simulink model "Model_6DOF_B3"  (R2020b)
settings: Solver=FixedStepAuto  StartTime=0.0  StopTime=120  FixedStep=0.05  RelTol=1e-3
values from neighbouring files (symbols this model uses):
  Ba_0 = [0 0 0 0 0 0]    [ctrl_mode_param.m]
  Bb = 4418825.3321    [load_data.m]
  Bv_0 = [tgt_speed 0 0 0 0 0]    [ctrl_mode_param.m]
  Bx_0 = [0 0 tgt_depth 0 0 0]    [ctrl_mode_param.m]
  Ixx = 5.23e7    (= 52300000)    [load_data.m]
  Ixy = 0    [load_data.m]
  Ixz = 0    [load_data.m]
  Iyy = 1.375e9    (= 1375000000)    [load_data.m]
  Iyz = 0    [load_data.m]
  Izz = 1.367e9    (= 1367000000)    [load_data.m]
  Mb = 4418825.3321    [load_data.m]
  Xb = 0    [load_data.m]
  Xg = 0    [load_data.m]
  Yb = 0    [load_data.m]
  Yg = 0    [load_data.m]
  Zb = 0.4406    [load_data.m]
  Zg = 0    [load_data.m]
undefined symbols (not defined in the file or in its folder): dA_BP1, dA_BP2, dA_Hull, dA_PH, dA_Sail, dA_SProot, dA_X1a, dA_X1b, dA_X2a, dA_X2b, dA_X3a, dA_X3b, dA_X4a, dA_X4b, its, n_BP1, n_BP2, n_Hull, n_PH, n_Sail, n_SProot, n_X1a, n_X1b, n_X2a, n_X2b, n_X3a, n_X3b, n_X4a, n_X4b, nt_BP1, nt_BP2, nt_Hull, nt_PH, nt_Sail, nt_SProot, nt_X1a, nt_X1b, nt_X2a, nt_X2b, nt_X3a, nt_X3b, nt_X4a, nt_X4b, Usp, vt1_BP1, vt1_BP2, vt1_Hull, vt1_PH, vt1_Sail, vt1_SProot, vt1_X1a, vt1_X1b, vt1_X2a, vt1_X2b, vt1_X3a, vt1_X3b, vt1_X4a, vt1_X4b, vt2_BP1, vt2_BP2 ... (+27)
libraries: simulink x5
(part 2 of 15)

== system Model_6DOF_B3/HDM 6DOF V1/M 6d org ==
  Bx : Inport
  Bv : Inport  Port=2
  Ba : Inport  Port=3
  Alpha : Inport  Port=4
  Umag : Inport  Port=5
  dX : Inport  Port=6
  UeX : Inport  Port=7
  dLCG : Inport  Port=8
  dmass : Inport  Port=9
  Mvm : Inport  Port=10
  M'prop : Lookup_n-D  NumberOfTableDimensions=1  BreakpointsForDimension1=[-7.7166666 -5.1444444 -3.08666664]  Table=[-0.00022 -0.0002 -0.00015]  InternalRulePriority=Speed  RndMeth=Simplest  InputSameDT=on
  M'uvw : Lookup_n-D  NumberOfTableDimensions=3  BreakpointsForDimension1=|  BreakpointsForDimension2=|  BreakpointsForDimension3=|  Table=|  InternalRulePriority=Speed  RndMeth=Simplest  InputSameDT=on
      BreakpointsForDimension1=|
      | [-12
      | -8
      | -4
      | 0
      | 4
      | 8
      | 12]
      BreakpointsForDimension2=|
      | [-5.1444E+00
      | -3.0866E+00
      | -1.5433E+00
      | ]
      Table=|
      | reshape([-2.40251E-03
      | -1.59538E-03
      | -8.21748E-04
      | -3.60182E-06
      | 8.13350E-04
      | 1.50586E-03
      | 2.39707E-03
      | -2.43392E-03
      | -1.61509E-03
      | -8.50748E-04
      | -3.60182E-06
      | 8.24271E-04
      | 1.51842E-03
      | 2.43805E-03
      | -2.45014E-03
      | -1.65711E-03
      | -9.11210E-04
      | -3.60182E-06
      | 8.61300E-04
      | 1.57459E-03
      | 2.42777E-03
      | -2.54380E-03
      | -1.68842E-03
      | -8.33041E-04
      | 2.23377E-05
      | 8.77717E-04
      | 1.73310E-03
      | 2.58847E-03
      | -2.63734E-03
      | -1.75078E-03
      | -8.64221E-04
      | 2.23377E-05
      | 9.08896E-04
      | 1.79546E-03
      | 2.68201E-03
      | -2.83738E-03
      | -1.88414E-03
      | -9.30902E-04
      | 2.23377E-05
      | 9.75577E-04
      | 1.92882E-03
      | 2.88206E-03
      | -2.63786E-03
      | -1.74504E-03
      | -8.52211E-04
      | 4.06140E-05
      | 9.33439E-04
      | 1.82626E-03
      | 2.71909E-03
      | -2.63728E-03
      | -1.74465E-03
      | -8.52017E-04
      | 4.06140E-05
      | 9.33245E-04
      | 1.82588E-03
      | 2.71851E-03
      | -2.86138E-03
      | -1.89405E-03
      | -9.26716E-04
      | 4.06140E-05
      | 1.00794E-03
      | 1.97527E-03
      | 2.94260E-03
      | -0.002723494
      | -0.001792522
      | -0.000861549
      | 6.9423E-05
      | 0.001000396
      | 0.001931368
      | 0.002862341
      | -0.002736476
      | -0.001798489
      | -0.000860502
      | 6.9423E-05
      | 0.001015473
      | 0.00195346
      | 0.002891447
      | -0.002765582
      | -0.00182058
      | -0.000875579
      | 6.9423E-05
      | 0.001014425
      | 0.001959426
      | 0.002904428],[7,3,4])
      BreakpointsForDimension3=|
      | [-35.0624 -18.3724 -15.3724 -13.8724
      | ]
      settings: InputPortMap=u0,u1,u2
  MATLAB Function2 : MATLAB Function  TreatAsAtomicUnit=on
  Mdxi : Subsystem
  Mqq2 : Lookup_n-D  NumberOfTableDimensions=1  BreakpointsForDimension1=|  Table=|  InternalRulePriority=Speed  RndMeth=Simplest  InputSameDT=on
      BreakpointsForDimension1=|
      | [-0.02
      | -0.015
      | -0.012958963
      | -0.009719222
      | -0.006479482
      | -0.003239741
      | -0.00161987
      | -0.000647948
      | 0.000647948
      | 0.00161987
      | 0.003239741
      | 0.006479482
      | 0.009719222
      | 0.012958963
      | 0.015
      | 0.02
      | ]
      Table=|
      | [-2.2571E-03
      | -2.3029E-03
      | -2.0965E-03
      | -2.0229E-03
      | -2.1546E-03
      | -1.4789E-03
      | -1.5664E-03
      | -1.4544E-03
      | -1.4705E-03
      | -1.4942E-03
      | -1.8790E-03
      | -1.8821E-03
      | -2.1009E-03
      | -2.0521E-03
      | -2.1685E-03
      | -2.0822E-03
      | ]
  Muq : Lookup_n-D  BreakpointsForDimension1=|  BreakpointsForDimension2=|  Table=|  InternalRulePriority=Speed  RndMeth=Simplest  InputSameDT=on
      BreakpointsForDimension1=|
      | [-2.00E-01
      | -1.50E-01
      | -1.00E-01
      | -5.00E-02
      | 0.00E+00
      | 5.00E-02
      | 1.00E-01
      | 1.50E-01
      | 2.00E-01
      | ]
      Table=|
      | reshape([-3.95902E-04
      | -2.96922E-04
      | -1.97952E-04
      | -9.89720E-05
      | 0.00000E+00
      | 9.89750E-05
      | 1.97948E-04
      | 2.96928E-04
      | 3.95898E-04
      | -4.94864E-04
      | -3.71144E-04
      | -2.47434E-04
      | -1.23714E-04
      | 0.00000E+00
      | 1.23715E-04
      | 2.47426E-04
      | 3.71146E-04
      | 4.94856E-04
      | -5.69298E-04
      | -4.26978E-04
      | -2.84648E-04
      | -1.42328E-04
      | 0.00000E+00
      | 1.42322E-04
      | 2.84652E-04
      | 4.26972E-04
      | 5.69302E-04
      | -5.60922E-04
      | -4.20692E-04
      | -2.80462E-04
      | -1.40232E-04
      | 0.00000E+00
      | 1.40228E-04
      | 2.80458E-04
      | 4.20688E-04
      | 5.60918E-04],[9,4])
      BreakpointsForDimension2=|
      | [-7.7166 -5.1444 -3.08664 -1.54332
      | ]
      settings: InputPortMap=u0,u1
  Mwq : Lookup_n-D  NumberOfTableDimensions=1  BreakpointsForDimension1=|  Table=|  InternalRulePriority=Speed  RndMeth=Simplest  InputSameDT=on
      BreakpointsForDimension1=|
      | [-0.0015
      | -0.0012
      | -0.0009
      | -0.0006
      | -0.0003
      | -0.0001
      | 0.0001
      | 0.0003
      | 0.0006
      | 0.0009
      | 0.0012
      | 0.0015]
      Table=|
      | [-1.3011E-02
      | -1.6962E-02
      | -2.0682E-02
      | -3.1419E-02
      | -6.4407E-02
      | -1.9322E-01
      | 1.9322E-01
      | 6.4378E-02
      | 3.1944E-02
      | 2.1072E-02
      | 1.6415E-02
      | 1.3407E-02]
  My : MATLAB Function  TreatAsAtomicUnit=on
  Product4 : Product
  Product5 : Product
  Saturation2 : Saturate  UpperLimit=0.0015  LowerLimit=-0.0015
  Saturation3 : Saturate  UpperLimit=0.02  LowerLimit=-0.02
  Selector10 : Selector  InputPortWidth=6  IndexOptions=Index vector (dialog)  Indices=1  OutputSizes=1
  Selector2 : Selector  InputPortWidth=6  IndexOptions=Index vector (dialog)  Indices=3  OutputSizes=1
  Selector4 : Selector  InputPortWidth=6  IndexOptions=Index vector (dialog)  Indices=5  OutputSizes=1
  Selector8 : Selector  InputPortWidth=6  IndexOptions=Index vector (dialog)  Indices=3  OutputSizes=1
  To Workspace : ToWorkspace  VariableName=MApp  SaveFormat=Timeseries  SampleTime=-1
  To Workspace1 : ToWorkspace  VariableName=MStat  SaveFormat=Timeseries  SampleTime=-1
  To Workspace2 : ToWorkspace  VariableName=MHull  SaveFormat=Timeseries  SampleTime=-1
  To Workspace3 : ToWorkspace  VariableName=Mprop  SaveFormat=Timeseries  SampleTime=-1
  To Workspace4 : ToWorkspace  VariableName=Mtotal  SaveFormat=Timeseries  SampleTime=-1
  M : Outport
  wires:
  Bv/1 -> Selector10/1, Selector4/1, Selector8/1, My/2(Bv)
  Bx/1 -> My/1(Bx), Selector2/1
  Selector10/1 -> Muq/2, Product4/1, M'uvw/2, M'prop/1
  Ba/1 -> My/3(Ba)
  M'prop/1 -> My/7(Mprop)
  UeX/1 -> My/10(UeX)
  Selector4/1 -> MATLAB Function2/1(u), Saturation3/1, Product4/2
  Alpha/1 -> M'uvw/1
  Umag/1 -> My/9(Umag)
  dLCG/1 -> My/11(dLCG)
  dmass/1 -> My/12(dmass)
  dX/1 -> Mdxi/1(dX)
  Mqq2/1 -> My/4(Mqq)
  Mwq/1 -> My/5(Mwq)
  Product4/1 -> Muq/1
  Product5/1 -> Saturation2/1
  Selector8/1 -> Product5/2
  MATLAB Function2/1(y) -> Product5/1
  Saturation2/1 -> Mwq/1
  Saturation3/1 -> Mqq2/1
  Muq/1 -> My/6(Muq)
  My/1(MY) -> To Workspace4/1, M/1
  Mdxi/1(MdX) -> My/13(MdXi)
  Mvm/1 -> My/14(Mvm)
  Selector2/1 -> M'uvw/3, Mdxi/2(z)
  M'uvw/1 -> My/8(Muvw)
  My/2(MYApp) -> To Workspace/1
  My/3(MYStat) -> To Workspace1/1
  My/5(MYprop) -> To Workspace3/1
  My/4(MYhull) -> To Workspace2/1

== system Model_6DOF_B3/HDM 6DOF V1/N ==
  Bx : Inport
  Bv : Inport  Port=2
  Ba : Inport  Port=3
  Beta : Inport  Port=4
  Umag : Inport  Port=5
  dX : Inport  Port=6
  UeX : Inport  Port=7
  dLCG : Inport  Port=8
  dmass : Inport  Port=9
  Nvm : Inport  Port=10
  Abs : Abs
  Abs1 : Abs
  Abs2 : Abs
  Gain : Gain  Gain=0.25
  Gain1 : Gain
  Mux : Mux
  Mz : MATLAB Function  TreatAsAtomicUnit=on
  N'r : Lookup_n-D  NumberOfTableDimensions=1  BreakpointsForDimension1=|  Table=|  InternalRulePriority=Speed  RndMeth=Simplest  InputSameDT=on
      BreakpointsForDimension1=|
      | [0.03999989
      | 0.079999993
      | 0.11999963
      | 0.15999956]
      Table=|
      | [-4.0344E-04
      | -8.1402E-04
      | -1.2116E-03
      | -1.6125E-03]
  N'r|r| : Lookup_n-D  NumberOfTableDimensions=1  BreakpointsForDimension1=|  Table=|  InternalRulePriority=Speed  RndMeth=Simplest  InputSameDT=on
      BreakpointsForDimension1=|
      | [-0.0015
      | -0.0012
      | -0.0009
      | -0.0006
      | -0.0003
      | -0.0001
      | 0.0001
      | 0.0003
      | 0.0006
      | 0.0009
      | 0.0012
      | 0.0015]
      Table=|
      | [-1.3011E-02
      | -1.6962E-02
      | -2.0682E-02
      | -3.1419E-02
      | -6.4407E-02
      | -1.9322E-01
      | 1.9322E-01
      | 6.4378E-02
      | 3.1944E-02
      | 2.1072E-02
      | 1.6415E-02
      | 1.3407E-02]
  N'uvw : Lookup_n-D  NumberOfTableDimensions=3  BreakpointsForDimension1=|  BreakpointsForDimension2=|  BreakpointsForDimension3=|  Table=|  InternalRulePriority=Speed  RndMeth=Simplest  InputSameDT=on
      BreakpointsForDimension1=|
      | [0
      | 4
      | 8
      | 12]
      BreakpointsForDimension2=|
      | [-5.1444E+00
      | -3.0866E+00
      | -1.5433E+00
      | ]
      Table=|
      | reshape([0.0000000E+00
      | 1.1975814E-03
      | 2.7970643E-03
      | 4.1308534E-03
      | 0.0000000E+00
      | 1.2111628E-03
      | 2.9207146E-03
      | 4.1207837E-03
      | 0.0000000E+00
      | 1.4959851E-03
      | 2.9486406E-03
      | 4.1213058E-03
      | 0.0000000E+00
      | 1.4879743E-03
      | 2.9975710E-03
      | 4.2577903E-03
      | 0.0000000E+00
      | 1.4933232E-03
      | 3.0017417E-03
      | 4.2334501E-03
      | 0.0000000E+00
      | 1.5365285E-03
      | 3.0446384E-03
      | 4.4091424E-03
      | 0.0000000E+00
      | 1.5329300E-03
      | 3.0664177E-03
      | 4.3937198E-03
      | 0.0000000E+00
      | 1.5274021E-03
      | 3.0742094E-03
      | 4.3066710E-03
      | 0.0000000E+00
      | 1.5692494E-03
      | 3.1052278E-03
      | 4.3211963E-03
      | 0.0000000E+00
      | 1.5996020E-03
      | 3.2227652E-03
      | 4.5425478E-03
      | 0.0000000E+00
      | 1.5650123E-03
      | 3.1236229E-03
      | 4.4022471E-03
      | 0.0000000E+00
      | 1.6041810E-03
      | 3.1241151E-03
      | 4.4103656E-03],[4,3,4])
      BreakpointsForDimension3=|
      | [-35.0624 -18.3724 -15.3724 -13.8724
      | ]
      settings: InputPortMap=u0,u1,u2
  N'vr : Lookup_n-D  NumberOfTableDimensions=1  BreakpointsForDimension1=|  Table=|  InternalRulePriority=Speed  RndMeth=Simplest  InputSameDT=on
      BreakpointsForDimension1=|
      | [-0.0015
      | -0.0012
      | -0.0009
      | -0.0006
      | -0.0003
      | -0.0001
      | 0.0001
      | 0.0003
      | 0.0006
      | 0.0009
      | 0.0012
      | 0.0015]
      Table=|
      | [-1.3011E-02
      | -1.6962E-02
      | -2.0682E-02
      | -3.1419E-02
      | -6.4407E-02
      | -1.9322E-01
      | 1.9322E-01
      | 6.4378E-02
      | 3.1944E-02
      | 2.1072E-02
      | 1.6415E-02
      | 1.3407E-02]
  NdXi : Subsystem
  Product{,1..2,4..5} (5 alike) : Product
  Scope2 : Scope
  Selector10 : Selector  InputPortWidth=6  IndexOptions=Index vector (dialog)  Indices=1  OutputSizes=1
  Selector2 : Selector  InputPortWidth=6  IndexOptions=Index vector (dialog)  Indices=3  OutputSizes=1
  Selector4 : Selector  InputPortWidth=6  IndexOptions=Index vector (dialog)  Indices=6  OutputSizes=1
  Selector8 : Selector  InputPortWidth=6  IndexOptions=Index vector (dialog)  Indices=2  OutputSizes=1
  Sign : Signum
  Sign1 : Signum
  N : Outport
  wires:
  Bv/1 -> Selector10/1, Selector4/1, Selector8/1, Mz/2(Bv)
  Bx/1 -> Mz/1(Bx), Selector2/1
  Selector10/1 -> N'uvw/2, Product1/1
  Ba/1 -> Mz/3(Ba)
  UeX/1 -> Mz/9(UeX)
  Beta/1 -> Sign1/1, Abs2/1
  Umag/1 -> Mz/8(Umag)
  dLCG/1 -> Mz/10(dLCG)
  dmass/1 -> Mz/11(dmass)
  dX/1 -> NdXi/1(dX)
  N'r/1 -> Product/2
  N'r|r|/1 -> Mz/5(CNrr)
  Product4/1 -> N'vr/1
  Selector8/1 -> Product4/1
  Abs/1 -> Product5/1
  Product5/1 -> N'r|r|/1
  Selector4/1 -> Product1/2, Product5/2, Abs/1, Product4/2
  N'vr/1 -> Mz/6(CNvr)
  Mz/1(N) -> N/1  "N Total"
  Selector2/1 -> NdXi/2(z), N'uvw/3
  N'uvw/1 -> Product2/2
  Product1/1 -> Sign/1, Abs1/1
  Abs1/1 -> N'r/1
  Sign/1 -> Product/1
  Product/1 -> Mz/4(CNr)
  Abs2/1 -> N'uvw/1
  Sign1/1 -> Product2/1
  Mz/3(NdX1) -> Mux/1
  Mz/4(NdX2) -> Mux/2
  Mz/5(NdX3) -> Mux/3
  Mz/6(NdX4) -> Mux/4
  Mux/1 -> Scope2/1
  Product2/1 -> Gain/1
  Gain/1 -> Mz/7(CNuvw)
  NdXi/1(NdXi) -> Gain1/1
  Gain1/1 -> Mz/12(CNdXi)
  Nvm/1 -> Mz/13(Nvm)

== system Model_6DOF_B3/HDM 6DOF V1/Wave Particle Velocity ==
  Bx_earth : Inport
  Bv_earth : Inport  Port=2
  Bv_ship : Inport  Port=3
  SeaState : Inport  Port=4
  dLCG : Inport  Port=5
  CG : Constant  Value=[32.3114 0 0]
  CGi : Constant  Value=|
      | [3.6451E+00 0.0000E+00 8.0728E-03; 9.8916E+00 0.0000E+00 2.5384E-01;
      | 1.6512E+01 0.0000E+00 3.0728E-01; 2.5395E+01 0.0000E+00 4.1417E-01; 3.4688E+01 0.0000E+00 4.1585E-01; 4.2324E+01 0.0000E+00 3.2444E-01; 4.9992E+01 0.0000E+00 3.3454E-01; 5.7427E+01 0.0000E+00 1.7420E-02; 6.3078E+01 0.0000E+00 1.8824E-02; 6.6703E+01 0.0000E+00 1.1340E-02; 2.5141E+01 0.0000E+00 8.6491E+00; 2.1732E+01 0.0000E+00 9.7273E+00; 6.3166E+01 0.0000E+00 -4.0823E-17; 2.2043E+01 0.0000E+00 9.7261E+00; 6.3451E+01 0.0000E+00 -6.2238E-17;]
  Cvm*dm Plateau : Constant  Value=|
      | [8.4658E+04	1.7229E+05	1.6487E+05
      | 2.3551E+04	4.3394E+05	3.6176E+05
      | 1.1585E+03	5.9767E+05	4.2996E+05
      | 1.4123E+02	1.1354E+06	6.5606E+05
      | 9.1503E+01	6.9712E+05	5.1688E+05
      | 9.6110E+01	6.7201E+05	5.1905E+05
      | 1.2163E+04	5.7818E+05	4.7547E+05
      | 3.7219E+04	3.4697E+05	3.3508E+05
      | 1.9318E+04	7.7284E+04	7.6560E+04
      | 1.5368E+04	2.6375E+04	2.6268E+04
      | 1.8312E+04	4.5870E+05	5.1108E+04
      | 3.1859E+02	1.2645E+04	3.4886E+02
      | 3.0285E+03	4.4945E+04	4.4489E+04
      | 7.9160E+02	8.8963E+02	1.3306E+04
      | 1.2115E+03	3.9547E+04	3.9205E+04
      | ]
  Demux : Demux  Outputs=3
  Demux1 : Demux  Outputs=3
  MATLAB Function : MATLAB Function  TreatAsAtomicUnit=on
  Mux : Mux  Inputs=6
  To Workspace1 : ToWorkspace  VariableName=VM_ForcesMoments  SaveFormat=Timeseries  SampleTime=-1
  Wave Particle Motions : Subsystem
  uws : Scope
  Xvm : Outport
  Yvm : Outport  Port=2
  Zvm : Outport  Port=3
  Kvm : Outport  Port=4
  Mvm : Outport  Port=5
  Nvm : Outport  Port=6
  z_eff : Outport  Port=7
  uwsXi : Outport  Port=8
  uwsCG : Outport  Port=9
  wires:
  Wave Particle Motions/4(zeff) -> z_eff/1
  Bx_earth/1 -> Wave Particle Motions/2(X_earth)
  Wave Particle Motions/2(ars) -> MATLAB Function/3(Ars)
  Wave Particle Motions/1(aws) -> MATLAB Function/2(Aws)
  CGi/1 -> Wave Particle Motions/3(CGi)
  CG/1 -> Wave Particle Motions/4(CG)
  Wave Particle Motions/3(Rs) -> MATLAB Function/4(Rs)
  SeaState/1 -> Wave Particle Motions/5(SeaState)
  dLCG/1 -> Wave Particle Motions/6(dLCG)
  Bv_ship/1 -> Wave Particle Motions/1(U_ship)
  MATLAB Function/7(Fvm) -> Demux/1  "Fvm"
  MATLAB Function/8(Mvm) -> Demux1/1  "Mvm"
  Demux/1 -> Xvm/1, Mux/1
  Demux/2 -> Yvm/1, Mux/2
  Demux/3 -> Zvm/1, Mux/3
  Demux1/2 -> Mux/5, Mvm/1
  Demux1/1 -> Kvm/1, Mux/4
  Demux1/3 -> Mux/6, Nvm/1
  Wave Particle Motions/5(uwXis) -> uwsXi/1
  Wave Particle Motions/6(uwsCG) -> uws/1, uwsCG/1
  Mux/1 -> To Workspace1/1
  Cvm*dm Plateau/1 -> MATLAB Function/1(cvm)

== system Model_6DOF_B3/HDM 6DOF V1/X ==
  Bx : Inport
  Bv : Inport  Port=2
  Ba : Inport  Port=3
  Umag : Inport  Port=4
  dXeff : Inport  Port=5
  UeSP : Inport  Port=6
  n : Inport  Port=7
  Alpha : Inport  Port=8
  dLCG : Inport  Port=9
  dmass : Inport  Port=10
  dXadd : Inport  Port=11
  dXraw : Inport  Port=12
  Xvm : Inport  Port=13
  Fx : MATLAB Function  TreatAsAtomicUnit=on
  Gain : Gain
  Gain20 : Gain  Gain=-1
  MATLAB Function2 : MATLAB Function  TreatAsAtomicUnit=on
  Mux : Mux  Inputs=6
  Product3 : Product
  Saturation1 : Saturate  UpperLimit=-1.543332  LowerLimit=-7.782
  Saturation2 : Saturate  UpperLimit=30  LowerLimit=-30
  Saturation3 : Saturate  UpperLimit=-1.54333333  LowerLimit=-5.1444
  Saturation6 : Saturate  UpperLimit=-1.543332  LowerLimit=-5.14444
  Saturation7 : Saturate  UpperLimit=-3.086664  LowerLimit=-7.71666
  Selector : Selector  InputPortWidth=6  IndexOptions=Index vector (dialog)  Indices=1  OutputSizes=1
  Selector1 : Selector  InputPortWidth=6  IndexOptions=Index vector (dialog)  Indices=3  OutputSizes=1
  Selector18 : Selector  InputPortWidth=6  IndexOptions=Index vector (dialog)  Indices=1  OutputSizes=1
  Selector19 : Selector  InputPortWidth=6  IndexOptions=Index vector (dialog)  Indices=1  OutputSizes=1
  Selector6 : Selector  InputPortWidth=6  IndexOptions=Index vector (dialog)  Indices=5  OutputSizes=1
  Subsystem1 : Subsystem
  T'wq : Lookup_n-D  BreakpointsForDimension1=|  BreakpointsForDimension2=|  Table=|  InternalRulePriority=Speed  RndMeth=Simplest  InputSameDT=on
      BreakpointsForDimension1=|
      | [-2.5000E-02
      | -2.0000E-02
      | -1.5000E-02
      | -1.0000E-02
      | -5.0000E-03
      | 0.0000E+00
      | 5.0000E-03
      | ]
      BreakpointsForDimension2=|
      | [-7.71666
      | -5.14444
      | -3.086664]
      Table=|
      | reshape([-2.7354E-04
      | -2.2597E-04
      | -1.7840E-04
      | -1.3083E-04
      | -8.3252E-05
      | -3.5680E-05
      | 1.1893E-05
      | -9.4081E-05
      | -7.5784E-05
      | -5.7487E-05
      | -3.9189E-05
      | -2.0892E-05
      | -2.5949E-06
      | 1.5702E-05
      | -1.4962E-04
      | -1.2035E-04
      | -9.1070E-05
      | -6.1795E-05
      | -3.2519E-05
      | -3.2436E-06
      | 2.6032E-05
      | ],[7,3])
      settings: InputPortMap=u0,u1
  "Thrust Deduction, 25m" : Lookup_n-D  NumberOfTableDimensions=1  BreakpointsForDimension1=[-5.14444,-3.086664,-1.543332]  BreakpointsForDimension2=[0.1 1.543332 3.086664 5.14444 100]  Table=[0.2496,0.2444134,0.245958]  InternalRulePriority=Speed  RndMeth=Simplest  InputSameDT=on
  To Workspace8 : ToWorkspace  VariableName=Benchmark_X  SaveFormat=Timeseries  SampleTime=-1
  Tprop : MATLAB Function  TreatAsAtomicUnit=on
  X'uvw : Lookup_n-D  BreakpointsForDimension1=|  BreakpointsForDimension2=|  Table=|  InternalRulePriority=Speed  RndMeth=Simplest  InputSameDT=on
      BreakpointsForDimension1=|
      | [-12
      | -8
      | -4
      | 0
      | 4
      | 8
      | 12]
      BreakpointsForDimension2=|
      | [-5.1444
      | -3.08664
      | -1.54332]
      Table=|
      | reshape([8.5556500E-04
      | 9.0045500E-04
      | 9.7379500E-04
      | 1.0292250E-03
      | 1.0286950E-03
      | 9.7963500E-04
      | 1.0147450E-03
      | 9.0637500E-04
      | 9.3710500E-04
      | 1.0133950E-03
      | 1.0723650E-03
      | 1.0693650E-03
      | 1.0284650E-03
      | 1.1084650E-03
      | 9.8653120E-04
      | 9.9350120E-04
      | 1.0534412E-03
      | 1.1098412E-03
      | 1.1115412E-03
      | 1.0836412E-03
      | 1.1582412E-03],[7,3])
      settings: InputPortMap=u0,u1
  X'wq : Lookup_n-D  BreakpointsForDimension1=|  BreakpointsForDimension2=[-7.71666 -5.14444 -3.086664 -1.543332]  Table=|  InternalRulePriority=Speed  RndMeth=Simplest  InputSameDT=on
      BreakpointsForDimension1=|
      | [-2.5000E-02
      | -2.0000E-02
      | -1.5000E-02
      | -1.0000E-02
      | -5.0000E-03
      | 0.0000E+00
      | 5.0000E-03
      | ]
      Table=|
      | reshape([2.0716E-04
      | 1.9060E-04
      | 1.7404E-04
      | 1.5748E-04
      | 1.4091E-04
      | 1.2435E-04
      | 1.0779E-04
      | 1.3610E-04
      | 1.1954E-04
      | 1.0298E-04
      | 8.6416E-05
      | 6.9855E-05
      | 5.3295E-05
      | 3.6734E-05
      | 1.5577E-04
      | 1.2817E-04
      | 1.0057E-04
      | 7.2967E-05
      | 4.5366E-05
      | 1.7765E-05
      | -9.8361E-06
      | 1.4245E-04
      | 1.1485E-04
      | 8.7244E-05
      | 5.9643E-05
      | 3.2042E-05
      | 4.4412E-06
      | -2.3160E-05
      | ],[7,4])
      settings: InputPortMap=u0,u1
  Xqq : Lookup_n-D  NumberOfTableDimensions=1  BreakpointsForDimension1=|  Table=|  InternalRulePriority=Speed  RndMeth=Simplest  InputSameDT=on
      BreakpointsForDimension1=|
      | [-0.02
      | -0.015
      | -0.012958963
      | -0.009719222
      | -0.006479482
      | -0.003239741
      | -0.00161987
      | -0.000647948
      | 0.000647948
      | 0.00161987
      | 0.003239741
      | 0.006479482
      | 0.009719222
      | 0.012958963
      | 0.015
      | 0.02
      | ]
      Table=|
      | [1.5581E-04
      | 1.1369E-04
      | 2.0348E-04
      | 4.5268E-04
      | 3.8456E-04
      | 9.9241E-05
      | 3.8998E-04
      | 9.1300E-05
      | -3.1574E-04
      | -7.9139E-05
      | -9.0517E-04
      | -4.4764E-04
      | -5.9612E-04
      | -5.5873E-04
      | -5.9343E-04
      | -5.5869E-04
      | ]
  rps : Scope
  thrus : Scope
  X : Outport
  wires:
  X'uvw/1 -> Fx/6(CXuvw)
  T'wq/1 -> Gain/1
  dXraw/1 -> Subsystem1/3(dX)
  dXeff/1 -> Subsystem1/4(dXeff)
  dXadd/1 -> Subsystem1/2(dXadd)
  Selector1/1 -> Product3/2
  Product3/1 -> X'wq/1, T'wq/1
  Selector18/1 -> Saturation1/1, Saturation7/1, Saturation6/1
  Subsystem1/1(Out1) -> Fx/12(XdXi)
  dmass/1 -> Fx/10(dmass)
  dLCG/1 -> Fx/9(dLCG)
  n/1 -> rps/1, Tprop/3(n_0)
  Ba/1 -> Fx/3(Ba)
  Bx/1 -> Fx/1(Bx)
  Saturation2/1 -> X'uvw/1
  Selector/1 -> Gain20/1
  Gain20/1 -> Tprop/1(speed)
  Fx/1(X) -> Mux/6, X/1
  Selector19/1 -> Saturation3/1
  Selector6/1 -> Product3/1, MATLAB Function2/1(u)
  Umag/1 -> Fx/8(Umag)
  MATLAB Function2/1(y) -> Xqq/1
  Alpha/1 -> Saturation2/1
  Bv/1 -> Selector6/1, Selector1/1, Selector18/1, Subsystem1/5(u), Selector/1, Selector19/1, Fx/2(Bv)
  Xqq/1 -> Fx/4(CXqq)
  Saturation3/1 -> "Thrust Deduction, 25m"/1
  "Thrust Deduction, 25m"/1 -> Tprop/2(Td)
  UeSP/1 -> Subsystem1/1(In1), Fx/11(UeSP)
  Tprop/1(Tprop) -> thrus/1, Fx/13(Tprop)
  Saturation1/1 -> X'wq/2
  Saturation6/1 -> X'uvw/2
  Saturation7/1 -> T'wq/2
  X'wq/1 -> Fx/5(CXwq)
  Xvm/1 -> Mux/5, Fx/14(Xvm)
  Gain/1 -> Fx/7(CTwq)
  Fx/2(Xapp) -> Mux/1
  Fx/3(Xhull) -> Mux/2
  Mux/1 -> To Workspace8/1
  Fx/9(X_Hyd) -> Mux/3
  Fx/4(Tout) -> Mux/4

== system Model_6DOF_B3/HDM 6DOF V1/X 6d org ==
  Bx : Inport
  Bv : Inport  Port=2
  Ba : Inport  Port=3
  Umag : Inport  Port=4
  dXeff : Inport  Port=5
  UeX : Inport  Port=6
  n : Inport  Port=7
  Alpha : Inport  Port=8
  dLCG : Inport  Port=9
  dmass : Inport  Port=10
  Xvm : Inport  Port=11
  Fx : MATLAB Function  TreatAsAtomicUnit=on
  Gain20 : Gain  Gain=-1
  MATLAB Function2 : MATLAB Function  TreatAsAtomicUnit=on
  Product3 : Product
  Saturation1 : Saturate  UpperLimit=-1  LowerLimit=-7.782
  Saturation2 : Saturate  UpperLimit=30  LowerLimit=-30
  Saturation3 : Saturate  UpperLimit=-1.54333333  LowerLimit=-7.782
  Selector : Selector  InputPortWidth=6  IndexOptions=Index vector (dialog)  Indices=1  OutputSizes=1
  Selector1 : Selector  InputPortWidth=6  IndexOptions=Index vector (dialog)  Indices=3  OutputSizes=1
  Selector18 : Selector  InputPortWidth=6  IndexOptions=Index vector (dialog)  Indices=1  OutputSizes=1
  Selector19 : Selector  InputPortWidth=6  IndexOptions=Index vector (dialog)  Indices=1  OutputSizes=1
  Selector2 : Selector  InputPortWidth=6  IndexOptions=Index vector (dialog)  Indices=3  OutputSizes=1
  Selector6 : Selector  InputPortWidth=6  IndexOptions=Index vector (dialog)  Indices=5  OutputSizes=1
  Subsystem1 : Subsystem
  T'wq : Lookup_n-D  BreakpointsForDimension1=|  BreakpointsForDimension2=|  Table=|  InternalRulePriority=Speed  RndMeth=Simplest  InputSameDT=on
      BreakpointsForDimension1=|
      | [-2.5000E-02
      | -2.0000E-02
      | -1.5000E-02
      | -1.0000E-02
      | -5.0000E-03
      | 0.0000E+00
      | 5.0000E-03
      | ]
      BreakpointsForDimension2=|
      | [-7.71666
      | -5.14444
      | -3.086664]
      Table=|
      | reshape([-2.7354E-04
      | -2.2597E-04
      | -1.7840E-04
      | -1.3083E-04
      | -8.3252E-05
      | -3.5680E-05
      | 1.1893E-05
      | -9.4081E-05
      | -7.5784E-05
      | -5.7487E-05
      | -3.9189E-05
      | -2.0892E-05
      | -2.5949E-06
      | 1.5702E-05
      | -1.4962E-04
      | -1.2035E-04
      | -9.1070E-05
      | -6.1795E-05
      | -3.2519E-05
      | -3.2436E-06
      | 2.6032E-05
      | ],[7,3])
      settings: InputPortMap=u0,u1
  "Thrust Deduction, 25m" : Lookup_n-D  NumberOfTableDimensions=1  BreakpointsForDimension1=[-5.14444,-3.086664,-1.543332]  BreakpointsForDimension2=[0.1 1.543332 3.086664 5.14444 100]  Table=[0.2496,0.2444134,0.245958]  InternalRulePriority=Speed  RndMeth=Simplest  InputSameDT=on
  To Workspace : ToWorkspace  VariableName=Xapp  SaveFormat=Timeseries  SampleTime=-1
  To Workspace1 : ToWorkspace  VariableName=Xstat  SaveFormat=Timeseries  SampleTime=-1
  To Workspace2 : ToWorkspace  VariableName=Xhull  SaveFormat=Timeseries  SampleTime=-1
  To Workspace3 : ToWorkspace  VariableName=Tout  SaveFormat=Timeseries  SampleTime=-1
  To Workspace4 : ToWorkspace  VariableName=Xtotal  SaveFormat=Timeseries  SampleTime=-1
  Tprop : MATLAB Function  TreatAsAtomicUnit=on
  X'uvw : Lookup_n-D  BreakpointsForDimension1=|  BreakpointsForDimension2=|  Table=|  InternalRulePriority=Speed  RndMeth=Simplest  InputSameDT=on
      BreakpointsForDimension1=|
      | [-12
      | -8
      | -4
      | 0
      | 4
      | 8
      | 12]
      BreakpointsForDimension2=|
      | [-5.1444
      | -3.08664
      | -1.54332]
      Table=|
      | reshape([8.0227E-04
      | 8.4716E-04
      | 9.2050E-04
      | 9.7593E-04
      | 9.7540E-04
      | 9.2634E-04
      | 9.6145E-04
      | 8.8861E-04
      | 9.1934E-04
      | 9.9563E-04
      | 1.0546E-03
      | 1.0516E-03
      | 1.0107E-03
      | 1.0907E-03
      | 9.8209E-04
      | 9.8906E-04
      | 1.0490E-03
      | 1.1054E-03
      | 1.1071E-03
      | 1.0792E-03
      | 1.1538E-03],[7,3])
      settings: InputPortMap=u0,u1
  X'wq : Lookup_n-D  BreakpointsForDimension1=|  BreakpointsForDimension2=[-7.71666 -5.14444 -3.086664 -1.543332]  Table=|  InternalRulePriority=Speed  RndMeth=Simplest  InputSameDT=on
      BreakpointsForDimension1=|
      | [-2.5000E-02
      | -2.0000E-02
      | -1.5000E-02
      | -1.0000E-02
      | -5.0000E-03
      | 0.0000E+00
      | 5.0000E-03
      | ]
      Table=|
      | reshape([2.0716E-04
      | 1.9060E-04
      | 1.7404E-04
      | 1.5748E-04
      | 1.4091E-04
      | 1.2435E-04
      | 1.0779E-04
      | 1.3610E-04
      | 1.1954E-04
      | 1.0298E-04
      | 8.6416E-05
      | 6.9855E-05
      | 5.3295E-05
      | 3.6734E-05
      | 1.5577E-04
      | 1.2817E-04
      | 1.0057E-04
      | 7.2967E-05
      | 4.5366E-05
      | 1.7765E-05
      | -9.8361E-06
      | 1.4245E-04
      | 1.1485E-04
      | 8.7244E-05
      | 5.9643E-05
      | 3.2042E-05
      | 4.4412E-06
      | -2.3160E-05
      | ],[7,4])
      settings: InputPortMap=u0,u1
  Xqq : Lookup_n-D  NumberOfTableDimensions=1  BreakpointsForDimension1=|  Table=|  InternalRulePriority=Speed  RndMeth=Simplest  InputSameDT=on
      BreakpointsForDimension1=|
      | [-0.02
      | -0.015
      | -0.012958963
      | -0.009719222
      | -0.006479482
      | -0.003239741
      | -0.00161987
      | -0.000647948
      | 0.000647948
      | 0.00161987
      | 0.003239741
      | 0.006479482
      | 0.009719222
      | 0.012958963
      | 0.015
      | 0.02
      | ]
      Table=|
      | [1.5581E-04
      | 1.1369E-04
      | 2.0348E-04
      | 4.5268E-04
      | 3.8456E-04
      | 9.9241E-05
      | 3.8998E-04
      | 9.1300E-05
      | -3.1574E-04
      | -7.9139E-05
      | -9.0517E-04
      | -4.4764E-04
      | -5.9612E-04
      | -5.5873E-04
      | -5.9343E-04
      | -5.5869E-04
      | ]
  X : Outport
  wires:
  Tprop/1(Tprop) -> Fx/13(Tprop)
  UeX/1 -> Subsystem1/1(UeX), Fx/11(UeX)
  "Thrust Deduction, 25m"/1 -> Tprop/2(Td)
  Saturation3/1 -> "Thrust Deduction, 25m"/1
  Xqq/1 -> Fx/4(CXqq)
  Bv/1 -> Selector19/1, Selector/1, Selector18/1, Selector1/1, Selector6/1, Fx/2(Bv)
  Alpha/1 -> Saturation2/1
  MATLAB Function2/1(y) -> Xqq/1
  Umag/1 -> Fx/8(Umag)
  Selector6/1 -> MATLAB Function2/1(u), Product3/1
  Selector19/1 -> Saturation3/1
  Fx/1(X) -> To Workspace4/1, X/1
  Gain20/1 -> Tprop/1(speed)
  Selector/1 -> Gain20/1
  Selector18/1 -> Saturation1/1
  Saturation2/1 -> X'uvw/1
  Bx/1 -> Fx/1(Bx), Selector2/1
  Ba/1 -> Fx/3(Ba)
  n/1 -> Tprop/3(n_0)
  dLCG/1 -> Fx/9(dLCG)
  dmass/1 -> Fx/10(dmass)
  Subsystem1/1(XdXi) -> Fx/12(XdXi)
  Saturation1/1 -> X'wq/2, X'uvw/2, T'wq/2
  Product3/1 -> X'wq/1, T'wq/1
  Selector1/1 -> Product3/2
  dXeff/1 -> Subsystem1/2(dXeff)
  X'wq/1 -> Fx/5(CXwq)
  T'wq/1 -> Fx/7(CTwq)
  X'uvw/1 -> Fx/6(CXuvw)
  Xvm/1 -> Fx/14(Xvm)
  Fx/2(Xapp) -> To Workspace/1
  Fx/3(Xstat) -> To Workspace1/1
  Fx/4(Xhull) -> To Workspace2/1
  Fx/5(Tout) -> To Workspace3/1
  Selector2/1 -> Subsystem1/3(z)

== system Model_6DOF_B3/HDM 6DOF V1/Y ==
  Bx : Inport
  Bv : Inport  Port=2
  Ba : Inport  Port=3
  Beta : Inport  Port=4
  Umag : Inport  Port=5
  dX : Inport  Port=6
  UeX : Inport  Port=7
  dLCG : Inport  Port=8
  dmass : Inport  Port=9
  Yvm : Inport  Port=10
  Abs1 : Abs
  Abs2 : Abs
  Fy : MATLAB Function  TreatAsAtomicUnit=on
  Gain2 : Gain
  Mux : Mux
  Product{,1..3} (4 alike) : Product
  Scope{,1..4} (5 alike) : Scope
  Selector2 : Selector  InputPortWidth=6  IndexOptions=Index vector (dialog)  Indices=6  OutputSizes=1
  Selector3 : Selector  InputPortWidth=6  IndexOptions=Index vector (dialog)  Indices=2  OutputSizes=1
  Selector4 : Selector  InputPortWidth=6  IndexOptions=Index vector (dialog)  Indices=3  OutputSizes=1
  Selector7 : Selector  InputPortWidth=6  IndexOptions=Index vector (dialog)  Indices=1  OutputSizes=1
  Sign : Signum
  Sign1 : Signum
  To Workspace : ToWorkspace  VariableName=Y_total  SaveFormat=Timeseries  SampleTime=-1
  To Workspace1 : ToWorkspace  VariableName=Y_ur  SaveFormat=Timeseries  SampleTime=-1
  To Workspace2 : ToWorkspace  VariableName=Yuvw  SaveFormat=Timeseries  SampleTime=-1
  To Workspace3 : ToWorkspace  VariableName=YdX  SaveFormat=Timeseries  SampleTime=-1
  To Workspace4 : ToWorkspace  VariableName=Y_app  SaveFormat=Timeseries  SampleTime=-1
  To Workspace5 : ToWorkspace  VariableName=Yhull  SaveFormat=Timeseries  SampleTime=-1
  Y'ur : Lookup_n-D  NumberOfTableDimensions=1  BreakpointsForDimension1=|  Table=|  InternalRulePriority=Speed  RndMeth=Simplest  InputSameDT=on
      BreakpointsForDimension1=|
      | [0.03999989
      | 0.079999993
      | 0.11999963
      | 0.15999956]
      Table=|
      | [-5.2094E-04
      | -1.0594E-03
      | -1.5649E-03
      | -2.0981E-03]
  Y'uvw : Lookup_n-D  NumberOfTableDimensions=3  BreakpointsForDimension1=|  BreakpointsForDimension2=|  BreakpointsForDimension3=|  Table=|  InternalRulePriority=Speed  RndMeth=Simplest  InputSameDT=on
      BreakpointsForDimension1=|
      | [0
      | 4
      | 8
      | 12]
      BreakpointsForDimension2=|
      | [-5.1444E+00
      | -3.0866E+00
      | -1.5433E+00
      | ]
      Table=|
      | reshape([0.0000000E+00
      | -5.0280621E-03
      | -9.4175348E-03
      | -1.4397458E-02
      | 0.0000000E+00
      | -5.0037454E-03
      | -9.1645405E-03
      | -1.4507402E-02
      | 0.0000000E+00
      | -4.2819107E-03
      | -9.0361786E-03
      | -1.4507235E-02
      | 0.0000000E+00
      | -4.7723270E-03
      | -9.7378407E-03
      | -1.5377541E-02
      | 0.0000000E+00
      | -4.7276301E-03
      | -9.6949815E-03
      | -1.5393721E-02
      | 0.0000000E+00
      | -4.5359209E-03
      | -9.4966039E-03
      | -1.6947859E-02
      | 0.0000000E+00
      | -5.1295007E-03
      | -1.0575377E-02
      | -1.6672924E-02
      | 0.0000000E+00
      | -4.9811404E-03
      | -1.0209461E-02
      | -1.6298327E-02
      | 0.0000000E+00
      | -4.7780219E-03
      | -1.0008968E-02
      | -1.6115181E-02
      | 0.0000000E+00
      | -5.7252015E-03
      | -1.1973447E-02
      | -1.9152812E-02
      | 0.0000000E+00
      | -5.2128737E-03
      | -1.0845978E-02
      | -1.7281669E-02
      | 0.0000000E+00
      | -4.9979037E-03
      | -1.0845685E-02
      | -1.6944141E-02],[4,3,4])
      BreakpointsForDimension3=|
      | [-35.0624 -18.3724 -15.3724 -13.8724
      | ]
      settings: InputPortMap=u0,u1,u2
  Y'|v|r : Lookup_n-D  NumberOfTableDimensions=1  BreakpointsForDimension1=|  Table=|  InternalRulePriority=Speed  RndMeth=Simplest  InputSameDT=on
      BreakpointsForDimension1=|
      | [-0.0015
      | -0.0012
      | -0.0009
      | -0.0006
      | -0.0003
      | -0.0001
      | 0.0001
      | 0.0003
      | 0.0006
      | 0.0009
      | 0.0012
      | 0.0015]
      Table=|
      | [-2.9784E-01
      | -2.6725E-01
      | -2.3292E-01
      | -2.0077E-01
      | -1.1489E-01
      | -7.6673E-03
      | -7.5516E-03
      | -1.1617E-01
      | -2.0077E-01
      | -2.9128E-01
      | -3.5974E-01
      | -4.7839E-01]
  YdXi : Subsystem
  Y|r|r : Lookup_n-D  NumberOfTableDimensions=1  BreakpointsForDimension1=|  Table=|  InternalRulePriority=Speed  RndMeth=Simplest  InputSameDT=on
      BreakpointsForDimension1=|
      | [-0.02
      | -0.015
      | -0.012958963
      | -0.009719222
      | -0.006479482
      | -0.003239741
      | -0.00161987
      | -0.000647948
      | 0.000647948
      | 0.00161987
      | 0.003239741
      | 0.006479482
      | 0.009719222
      | 0.012958963
      | 0.015
      | 0.02
      | ]
      Table=|
      | [3.6478E-03
      | 3.8686E-03
      | 3.4313E-03
      | 4.0790E-03
      | 3.9500E-03
      | 3.6018E-03
      | 3.6796E-03
      | 3.5502E-03
      | 3.4310E-03
      | 3.4872E-03
      | 4.2239E-03
      | 4.0934E-03
      | 3.0314E-03
      | 2.5726E-03
      | 2.9188E-03
      | 2.7740E-03
      | ]
  Y : Outport
  wires:
  Selector7/1 -> Product3/2, Y'uvw/2
  Beta/1 -> Scope3/1, Sign/1, Abs1/1
  Bv/1 -> Selector7/1, Selector3/1, Selector2/1, Fy/2(Bv)
  Umag/1 -> Fy/8(Umag)
  Bx/1 -> Selector4/1, Fy/1(Bx)
  UeX/1 -> Fy/9(UeX)
  Selector3/1 -> Product1/2
  Ba/1 -> Fy/3(Ba)
  dLCG/1 -> Fy/10(dLCG)
  dmass/1 -> Fy/11(dmass)
  dX/1 -> Scope/1, YdXi/1(dX)
  Product3/1 -> Abs2/1, Sign1/1
  Product1/1 -> Y'|v|r/1
  Selector2/1 -> Product1/1, Product3/1, Y|r|r/1
  Y'|v|r/1 -> Fy/6(CYrr)
  Fy/1(Fy) -> Y/1, To Workspace/1, Scope1/1
  Y|r|r/1 -> Fy/4(CYr)
  Y'ur/1 -> Product2/2
  Selector4/1 -> YdXi/2(z), Y'uvw/3
  Y'uvw/1 -> Product/2
  Sign/1 -> Product/1
  Abs1/1 -> Y'uvw/1
  Product2/1 -> Fy/5(CYvr)
  Sign1/1 -> Product2/1
  Abs2/1 -> Y'ur/1
  Fy/2(FYr) -> To Workspace1/1
  Fy/7(FYuvw) -> To Workspace2/1
  Fy/3(FYx1) -> Mux/1
  Fy/4(FYx2) -> Mux/2
  Fy/5(FYx3) -> Mux/3
  Fy/6(FYx4) -> Mux/4
  Mux/1 -> To Workspace3/1
  Fy/8(FYhull) -> To Workspace5/1
  YdXi/1(YdX) -> Scope4/1, Fy/12(CYdXi)
  Product/1 -> Gain2/1
  Gain2/1 -> Scope2/1, Fy/7(CYuvw)
  Fy/9(FYApp) -> To Workspace4/1
  Yvm/1 -> Fy/13(Yvm)

== system Model_6DOF_B3/HDM 6DOF V1/Z ==
  Bx : Inport
  Bv : Inport  Port=2
  Ba : Inport  Port=3
  Alpha : Inport  Port=4
  Umag : Inport  Port=5
  dX : Inport  Port=6
  UeSP : Inport  Port=7
  dLCG : Inport  Port=8
  dmass : Inport  Port=9
  Zvm : Inport  Port=10
  Fz : MATLAB Function  TreatAsAtomicUnit=on
  Gain : Gain
  Gain1 : Gain  Gain=0.7
  MATLAB Function : MATLAB Function  TreatAsAtomicUnit=on
  Mux : Mux  Inputs=6
  Product1 : Product
  Product3 : Product
  Saturation1 : Saturate  UpperLimit=0.04  LowerLimit=-0.04
  Saturation2 : Saturate  UpperLimit=0.0015  LowerLimit=-0.0015
  Saturation3 : Saturate  UpperLimit=0.02  LowerLimit=-0.02
  Saturation4 : Saturate  UpperLimit=-13.8724  LowerLimit=-35.0624
  Selector2 : Selector  InputPortWidth=6  IndexOptions=Index vector (dialog)  Indices=5  OutputSizes=1
  Selector3 : Selector  InputPortWidth=6  IndexOptions=Index vector (dialog)  Indices=3  OutputSizes=1
  Selector4 : Selector  InputPortWidth=6  IndexOptions=Index vector (dialog)  Indices=3  OutputSizes=1
  Selector7 : Selector  InputPortWidth=6  IndexOptions=Index vector (dialog)  Indices=1  OutputSizes=1
  To Workspace8 : ToWorkspace  VariableName=Benchmark_Z  SaveFormat=Timeseries  SampleTime=-1
  Z'uq Prop : Lookup_n-D  BreakpointsForDimension1=|  BreakpointsForDimension2=[-7.71666 -5.14444 -3.086664 -1.543332]  Table=|  InternalRulePriority=Speed  RndMeth=Simplest  InputSameDT=on
      BreakpointsForDimension1=|
      | [-2.0E-01
      | -1.5E-01
      | -1.0E-01
      | -5.0E-02
      | 0.0E+00
      | 5.0E-02
      | 1.0E-01
      | 1.5E-01
      | 2.0E-01
      | ]
      Table=|
      | reshape([1.3913E-04
      | 1.0452E-04
      | 6.9900E-05
      | 3.5283E-05
      | 6.6700E-07
      | -3.3949E-05
      | -6.8566E-05
      | -1.0318E-04
      | -1.3780E-04
      | 2.8914E-04
      | 2.1702E-04
      | 1.4490E-04
      | 7.2785E-05
      | 6.6700E-07
      | -7.1451E-05
      | -1.4357E-04
      | -2.1569E-04
      | -2.8780E-04
      | 1.1606E-04
      | 8.7208E-05
      | 5.8361E-05
      | 2.9514E-05
      | 6.6700E-07
      | -2.8180E-05
      | -5.7027E-05
      | -8.5874E-05
      | -1.1472E-04
      | 1.1606E-04
      | 8.7208E-05
      | 5.8361E-05
      | 2.9514E-05
      | 6.6700E-07
      | -2.8180E-05
      | -5.7027E-05
      | -8.5874E-05
      | -1.1472E-04],[9,4])
      settings: InputPortMap=u0,u1
  Z'uvw1 : Lookup_n-D  NumberOfTableDimensions=3  BreakpointsForDimension1=|  BreakpointsForDimension2=|  BreakpointsForDimension3=|  Table=|  InternalRulePriority=Speed  RndMeth=Simplest  InputSameDT=on
      BreakpointsForDimension1=|
      | [-12
      | -8
      | -4
      | 0
      | 4
      | 8
      | 12]
      BreakpointsForDimension2=|
      | [-5.1444E+00
      | -3.0866E+00
      | -1.5433E+00
      | ]
      Table=|
      | reshape([-3.82587E-03
      | -2.42543E-03
      | -1.05453E-03
      | 1.94202E-04
      | 1.48991E-03
      | 3.04047E-03
      | 4.14104E-03
      | -3.76348E-03
      | -2.38508E-03
      | -9.82619E-04
      | 1.94202E-04
      | 1.47560E-03
      | 3.02863E-03
      | 4.06663E-03
      | -3.75964E-03
      | -2.29001E-03
      | -8.34074E-04
      | 1.94202E-04
      | 1.38956E-03
      | 2.91153E-03
      | 4.15251E-03
      | -3.11218E-03
      | -1.80502E-03
      | -4.97855E-04
      | 8.09305E-04
      | 2.11647E-03
      | 3.42363E-03
      | 4.73079E-03
      | -2.62573E-03
      | -1.48072E-03
      | -3.35708E-04
      | 8.09305E-04
      | 1.95432E-03
      | 3.09933E-03
      | 4.24434E-03
      | -2.06413E-03
      | -1.10632E-03
      | -1.48507E-04
      | 8.09305E-04
      | 1.76712E-03
      | 2.72493E-03
      | 3.68274E-03
      | -3.09997E-03
      | -1.76300E-03
      | -4.26025E-04
      | 9.10947E-04
      | 2.24792E-03
      | 3.58489E-03
      | 4.92186E-03
      | -2.49055E-03
      | -1.35672E-03
      | -2.22886E-04
      | 9.10947E-04
      | 2.04478E-03
      | 3.17861E-03
      | 4.31245E-03
      | -2.64104E-03
      | -1.45704E-03
      | -2.73048E-04
      | 9.10947E-04
      | 2.09494E-03
      | 3.27894E-03
      | 4.46293E-03
      | -0.003059752
      | -0.001711935
      | -0.000364117
      | 0.0009837
      | 0.002331518
      | 0.003679335
      | 0.005027153
      | -0.002351082
      | -0.0012256
      | -0.000100118
      | 0.0009837
      | 0.002109182
      | 0.003234664
      | 0.004360146
      | -0.001725739
      | -0.000822593
      | 8.05539E-05
      | 0.0009837
      | 0.001886847
      | 0.002789993
      | 0.00369314],[7,3,4])
      BreakpointsForDimension3=|
      | [-35.0624 -18.3724 -15.3724 -13.8724
      | ]
      settings: InputPortMap=u0,u1,u2
  ZdXi : Subsystem
  Zqq : Lookup_n-D  NumberOfTableDimensions=1  BreakpointsForDimension1=|  Table=|  InternalRulePriority=Speed  RndMeth=Simplest  InputSameDT=on
      BreakpointsForDimension1=|
      | [-0.02
      | -0.015
      | -0.012958963
      | -0.009719222
      | -0.006479482
      | -0.003239741
      | -0.00161987
      | -0.000647948
      | 0.000647948
      | 0.00161987
      | 0.003239741
      | 0.006479482
      | 0.009719222
      | 0.012958963
      | 0.015
      | 0.02
      | ]
      Table=|
      | [3.6478E-03
      | 3.8686E-03
      | 3.4313E-03
      | 4.0790E-03
      | 3.9500E-03
      | 3.6018E-03
      | 3.6796E-03
      | 3.5502E-03
      | 3.4310E-03
      | 3.4872E-03
      | 4.2239E-03
      | 4.0934E-03
      | 3.0314E-03
      | 2.5726E-03
      | 2.9188E-03
      | 2.7740E-03
      | ]
  Zuq : Lookup_n-D  NumberOfTableDimensions=1  BreakpointsForDimension1=|  Table=|  InternalRulePriority=Speed  RndMeth=Simplest  InputSameDT=on
      BreakpointsForDimension1=|
      | [-0.04
      | -0.03
      | -0.02
      | -0.01
      | -0.005
      | -0.002
      | 0.002
      | 0.005
      | 0.01
      | 0.02
      | 0.03
      | 0.04
      | ]
      Table=|
      | [-9.8908E-03
      | -9.0784E-03
      | -8.9566E-03
      | -1.0733E-02
      | -1.4141E-02
      | -2.4189E-02
      | -6.5605E-03
      | -7.1594E-03
      | -7.6366E-03
      | -7.9008E-03
      | -6.1794E-03
      | -6.1029E-03
      | ]
  Zwq : Lookup_n-D  NumberOfTableDimensions=1  BreakpointsForDimension1=|  Table=|  InternalRulePriority=Speed  RndMeth=Simplest  InputSameDT=on
      BreakpointsForDimension1=|
      | [-0.0015
      | -0.0012
      | -0.0009
      | -0.0006
      | -0.0003
      | -0.0001
      | 0.0001
      | 0.0003
      | 0.0006
      | 0.0009
      | 0.0012
      | 0.0015]
      Table=|
      | [-2.9784E-01
      | -2.6725E-01
      | -2.3292E-01
      | -2.0077E-01
      | -1.1489E-01
      | -7.6673E-03
      | -7.5516E-03
      | -1.1617E-01
      | -2.0077E-01
      | -2.9128E-01
      | -3.5974E-01
      | -4.7839E-01]
  Z : Outport
  wires:
  Z'uvw1/1 -> Gain/1
  Selector4/1 -> Saturation4/1
  Zvm/1 -> Mux/5, Fz/14(Zvm)
  Ba/1 -> Fz/3(Ba)
  ZdXi/1(ZdX) -> Fz/13(ZdXi)
  Zuq/1 -> Fz/5(Zuq)
  Fz/1(Fz) -> Mux/6, Z/1
  Saturation3/1 -> Zqq/1
  Saturation2/1 -> Zwq/1
  Saturation1/1 -> Zuq/1
  dX/1 -> ZdXi/1(dX)
  dmass/1 -> Fz/12(dmass)
  dLCG/1 -> Fz/11(dLCG)
  Product1/1 -> Saturation2/1
  Selector3/1 -> Product1/2
  UeSP/1 -> Fz/10(UeSP)
  Product3/1 -> Z'uq Prop/1, Saturation1/1
  Bx/1 -> Selector4/1, Fz/1(Bx)
  Umag/1 -> Fz/9(Umag)
  Bv/1 -> Selector2/1, Selector3/1, Selector7/1, Fz/2(Bv)
  Alpha/1 -> MATLAB Function/1(x), Z'uvw1/1
  Selector2/1 -> Product3/1, Saturation3/1, Product1/1
  Selector7/1 -> Product3/2, Z'uq Prop/2, Z'uvw1/2
  Zwq/1 -> Fz/6(Zwq)
  Z'uq Prop/1 -> Fz/8(CZProp)
  Zqq/1 -> Fz/4(Zqq)
  Saturation4/1 -> Z'uvw1/3, ZdXi/2(z)
  Gain/1 -> ?
  MATLAB Function/1(y) -> Gain1/1
  Gain1/1 -> Fz/7(Zuvw)
  Mux/1 -> To Workspace8/1
  Fz/2(FZApp) -> Mux/1
  Fz/4(FZHull) -> Mux/2
  Fz/7(FZ_Hyd) -> Mux/3
  Fz/5(FZProp) -> Mux/4
